simulink model "sg_lens_correct"  (Simulink 8.2)
settings: Solver=VariableStepDiscrete  StartTime=0.0  StopTime=3*Npxl  RelTol=1e-3
values from neighbouring files (symbols this model uses):
  ImgStrmIn = ImgDist'    [tb_lens_correct.m]
  ImgX = SizeI(2)    [tb_lens_correct.m]
  ImgY = SizeI(1)    [tb_lens_correct.m]
  IPM = 0    [tb_lens_correct.m]
  K = 0.00004    (= 4e-05)    [tb_lens_correct.m]
  Npxl = ImgY * ImgX    [tb_lens_correct.m]
  Radius_ROM = Radius'    [tb_lens_correct.m]
  Xcent = (ImgX-1)/2    [tb_lens_correct.m]
  Ycent = (ImgY-1)/2    [tb_lens_correct.m]
libraries: xbsIndex_r4 x87, dspsrcs4 x3
settings Model: Creator=sps  LastModifiedBy=tawassne
settings OptimizationCC: InitFltsAndDblsToZero=on
settings DebuggingCC: SaveWithParameterizedLinksMsg=none  SignalResolutionControl=TryResolveAllWithWarning  SolverPrmCheckMsg=none  MultiTaskDSMMsg=warning  MultiTaskCondExecSysMsg=none
settings RTWCC: IncludeERTFirstTime=on
settings GRTTargetCC: TargetFcnLib=ansi_tfl_tmw.mat

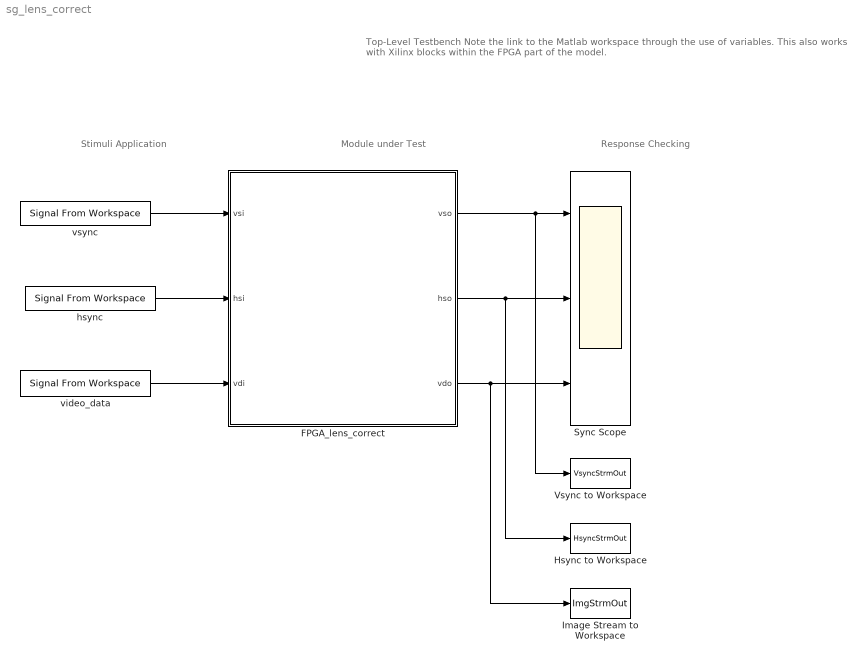
== system sg_lens_correct ==
  note: Top-Level Testbench
      | Note the link to the Matlab workspace through the use of variables.
      | This also works with Xilinx blocks within the FPGA part of the model.
  note: Stimuli Application
  note: Response Checking
  note: Module under Test
  FPGA_lens_correct : Subsystem
  Hsync to Workspace : ToWorkspace  VariableName=HsyncStrmOut  SampleTime=-1
      settings: MaxDataPoints=2*Npxl
  Image Stream to Workspace : ToWorkspace  VariableName=ImgStrmOut  SampleTime=-1
      settings: MaxDataPoints=2*Npxl
  Sync Scope : Scope  NumInputPorts=3
      settings: YMin=-5~-5~-5  YMax=5~5~5
  Vsync to Workspace : ToWorkspace  VariableName=VsyncStrmOut  SampleTime=-1
      settings: MaxDataPoints=2*Npxl
  hsync : dspsrcs4/Signal From Workspace  X=[ zeros(1,ImgX-1) 1 ]  Ts=1  nsamps=1  OutputAfterFinalValue=Cyclic repetition  ignoreOrWarnInputAndFrameLengths=off
  video_data : dspsrcs4/Signal From Workspace  X=[ ImgStrmIn(:) ]  Ts=1  nsamps=1  OutputAfterFinalValue=Cyclic repetition  ignoreOrWarnInputAndFrameLengths=off
  vsync : dspsrcs4/Signal From Workspace  X=[ zeros(1,Npxl-1) 1 ]  Ts=1  nsamps=1  OutputAfterFinalValue=Cyclic repetition  ignoreOrWarnInputAndFrameLengths=off
  wires:
  vsync/1 -> FPGA_lens_correct/1(vsi)
  hsync/1 -> FPGA_lens_correct/2(hsi)
  video_data/1 -> FPGA_lens_correct/3(vdi)
  FPGA_lens_correct/1(vso) -> Sync Scope/1, Vsync to Workspace/1
  FPGA_lens_correct/2(hso) -> Sync Scope/2, Hsync to Workspace/1
  FPGA_lens_correct/3(vdo) -> Sync Scope/3, Image Stream to Workspace/1

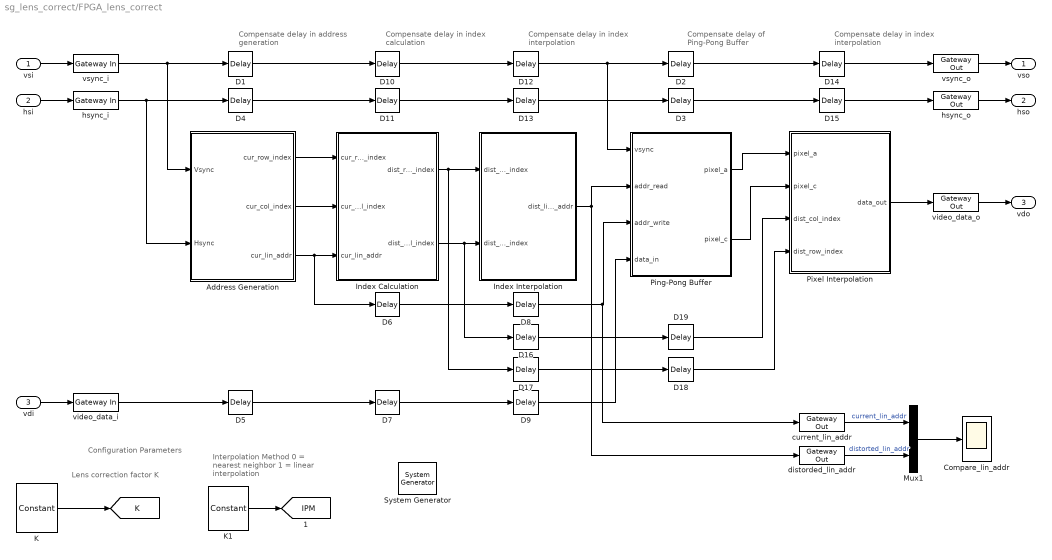
== system sg_lens_correct/FPGA_lens_correct ==
  note: Compensate delay
      | of Ping-Pong Buffer
  note: Compensate delay
      | in index calculation
  note: Compensate delay
      | in index interpolation
  note: Compensate delay
      | in address generation
  note: Configuration Parameters
  note: Lens correction factor K
  note: Interpolation Method
      | 0 = nearest neighbor
      | 1 = linear interpolation
  note: Compensate delay
      | in index interpolation
  vsi : Inport
  hsi : Inport  Port=2
  vdi : Inport  Port=3
  " System Generator" : xbsIndex_r4/ System Generator  Tag=genX  xilinxfamily=spartan6  part=xc6slx150t  speed=-3  package=fgg676  synthesis_tool=XST  clock_wrapper=Clock Enables  directory=./sg_gamma_s6  proj_type=Project Navigator  Synth_file=XST Defaults  Impl_file=ISE Defaults  testbench=off  simulink_period=1  sysclk_period=10  dcm_input_clock_period=10  incr_netlist=off  trim_vbits=Everywhere in SubSystem  dbl_ovrd=According to Block Masks  core_generation=According to Block Masks  run_coregen=off  deprecated_control=off  eval_field=0  block_type=sysgen
      settings: block_version=11.4
  Address Generation : Subsystem
  Compare_lin_addr : Scope
      settings: ShowLegends=on  SaveName=ScopeData3
  D1 : xbsIndex_r4/Delay  rst=off  infoeditControl=Selection of Reset will increase slice count due to use of real FFs and instead of SRLs  en=off  latency=LT_AdrGen  dbl_ovrd=off  reg_retiming=off  block_type=delay
  D{6..7,10..11} (4 alike) : xbsIndex_r4/Delay  rst=off  infoeditControl=Selection of Reset will increase slice count due to use of real FFs and instead of SRLs  en=off  latency=LT_IdxCalc  dbl_ovrd=off  reg_retiming=off  block_type=delay
  D{8..9,12..13,16..17} (6 alike) : xbsIndex_r4/Delay  rst=off  infoeditControl=Selection of Reset will increase slice count due to use of real FFs and instead of SRLs  en=off  latency=LT_IdxInpol  dbl_ovrd=off  reg_retiming=off  block_type=delay
  D14 : xbsIndex_r4/Delay  rst=off  infoeditControl=Selection of Reset will increase slice count due to use of real FFs and instead of SRLs  en=off  latency=LT_PxlInpol  dbl_ovrd=off  reg_retiming=off  block_type=delay
  D15 : xbsIndex_r4/Delay  rst=off  infoeditControl=Selection of Reset will increase slice count due to use of real FFs and instead of SRLs  en=off  latency=LT_PxlInpol  dbl_ovrd=off  reg_retiming=off  block_type=delay
  D{2..3,18..19} (4 alike) : xbsIndex_r4/Delay  rst=off  infoeditControl=Selection of Reset will increase slice count due to use of real FFs and instead of SRLs  en=off  latency=LT_PingPong  dbl_ovrd=off  reg_retiming=off  block_type=delay
  D4 : xbsIndex_r4/Delay  rst=off  infoeditControl=Selection of Reset will increase slice count due to use of real FFs and instead of SRLs  en=off  latency=LT_AdrGen  dbl_ovrd=off  reg_retiming=off  block_type=delay
  D5 : xbsIndex_r4/Delay  rst=off  infoeditControl=Selection of Reset will increase slice count due to use of real FFs and instead of SRLs  en=off  latency=LT_AdrGen  dbl_ovrd=off  reg_retiming=off  block_type=delay
  Index Calculation : Subsystem
  Index Interpolation : Subsystem
  K : xbsIndex_r4/Constant  const=K  gui_display_data_type=Fixed-point  arith_type=Unsigned  n_bits=32  bin_pt=31  preci_type=Single  exp_width=8  frac_width=24  explicit_period=off  period=1  equ=P=C  opselect=C  inp2=PCIN>>17  opr=+  inp1=P  carry=CIN  dbl_ovrd=off  block_type=constant
  K1 : xbsIndex_r4/Constant  const=IPM  gui_display_data_type=Boolean  arith_type=Boolean  n_bits=16  bin_pt=15  preci_type=Single  exp_width=8  frac_width=24  explicit_period=off  period=1  equ=P=C  opselect=C  inp2=PCIN>>17  opr=+  inp1=P  carry=CIN  dbl_ovrd=off  block_type=constant
  Mux1 : Mux  Inputs=2
  Ping-Pong Buffer : Subsystem
  Pixel Interpolation : Subsystem
  current_lin_addr : xbsIndex_r4/Gateway Out  hdl_port=off  timing_constraint=None  locs_specified=off  LOCs={}  block_type=gatewayout
      settings: infoedit="Gateway out block.  Converts Xilinx fixed point or floating-point type inputs into ouputs of type Simulink integer, double, or fixed point.<br><br>Hardware notes:  In hardware these blocks become top level output ports or are discarded, depending on how they are configured."  xl_area=[0, 0, 0, 0, 0, 0, 0]  block_version=VER_STRING_GOES_HERE
  distorded_lin_addr : xbsIndex_r4/Gateway Out  hdl_port=off  timing_constraint=None  locs_specified=off  LOCs={}  block_type=gatewayout
      settings: infoedit="Gateway out block.  Converts Xilinx fixed point or floating-point type inputs into ouputs of type Simulink integer, double, or fixed point.<br><br>Hardware notes:  In hardware these blocks become top level output ports or are discarded, depending on how they are configured."  xl_area=[0, 0, 0, 0, 0, 0, 0]  block_version=VER_STRING_GOES_HERE
  hsync_i : xbsIndex_r4/Gateway In  gui_display_data_type=Fixed-point  arith_type=Boolean  n_bits=1  bin_pt=0  preci_type=Single  exp_width=8  frac_width=24  quantization="Round  (unbiased: +/- Inf)"  overflow=Saturate  period=1  dbl_ovrd=off  timing_constraint=None  locs_specified=off  LOCs={}  hdl_port=on  block_type=gatewayin
      settings: infoedit="Gateway in block.  Converts inputs of type Simulink integer, double and fixed point to  Xilinx fixed point type.<br><br>Hardware notes:  In hardware these blocks become top level input ports."  xl_area=[0, 0, 0, 0, 0, 0, 0]  block_version=VER_STRING_GOES_HERE
  hsync_o : xbsIndex_r4/Gateway Out  hdl_port=on  timing_constraint=None  locs_specified=off  LOCs={}  block_type=gatewayout
      settings: infoedit="Gateway out block.  Converts Xilinx fixed point inputs into ouputs of type Simulink integer, double, or fixed point.<P><P>Hardware notes:  In hardware these blocks become top level output ports or are discarded, depending on how they are configured."  xl_area=[0, 0, 0, 0, 0, 0, 0]  block_version=VER_STRING_GOES_HERE
  video_data_i : xbsIndex_r4/Gateway In  gui_display_data_type=Fixed-point  arith_type=Unsigned  n_bits=8  bin_pt=0  preci_type=Single  exp_width=8  frac_width=24  quantization="Round  (unbiased: +/- Inf)"  overflow=Saturate  period=1  dbl_ovrd=off  timing_constraint=None  locs_specified=off  LOCs={}  hdl_port=on  block_type=gatewayin
      settings: infoedit="Gateway in block.  Converts inputs of type Simulink integer, double and fixed point to  Xilinx fixed point type.<br><br>Hardware notes:  In hardware these blocks become top level input ports."  xl_area=[0, 0, 0, 0, 0, 0, 0]  block_version=VER_STRING_GOES_HERE
  video_data_o : xbsIndex_r4/Gateway Out  hdl_port=on  timing_constraint=None  locs_specified=off  LOCs={}  block_type=gatewayout
      settings: infoedit="Gateway out block.  Converts Xilinx fixed point inputs into ouputs of type Simulink integer, double, or fixed point.<P><P>Hardware notes:  In hardware these blocks become top level output ports or are discarded, depending on how they are configured."  xl_area=[0, 0, 0, 0, 0, 0, 0]  block_version=VER_STRING_GOES_HERE
  vsync_i : xbsIndex_r4/Gateway In  gui_display_data_type=Fixed-point  arith_type=Boolean  n_bits=1  bin_pt=0  preci_type=Single  exp_width=8  frac_width=24  quantization="Round  (unbiased: +/- Inf)"  overflow=Saturate  period=1  dbl_ovrd=off  timing_constraint=None  locs_specified=off  LOCs={}  hdl_port=on  block_type=gatewayin
      settings: infoedit="Gateway in block.  Converts inputs of type Simulink integer, double and fixed point to  Xilinx fixed point type.<br><br>Hardware notes:  In hardware these blocks become top level input ports."  xl_area=[0, 0, 0, 0, 0, 0, 0]  block_version=VER_STRING_GOES_HERE
  vsync_o : xbsIndex_r4/Gateway Out  hdl_port=on  timing_constraint=None  locs_specified=off  LOCs={}  block_type=gatewayout
      settings: infoedit="Gateway out block.  Converts Xilinx fixed point inputs into ouputs of type Simulink integer, double, or fixed point.<P><P>Hardware notes:  In hardware these blocks become top level output ports or are discarded, depending on how they are configured."  xl_area=[0, 0, 0, 0, 0, 0, 0]  block_version=VER_STRING_GOES_HERE
  vso : Outport
  hso : Outport  Port=2
  vdo : Outport  Port=3
  tag scope: IPM=global, K=global
  wires:
  vdi/1 -> video_data_i/1
  video_data_o/1 -> vdo/1
  vsi/1 -> vsync_i/1
  hsi/1 -> hsync_i/1
  vsync_o/1 -> vso/1
  hsync_o/1 -> hso/1
  vsync_i/1 -> Address Generation/1(Vsync), D1/1
  hsync_i/1 -> Address Generation/2(Hsync), D4/1
  Address Generation/3(cur_lin_addr) -> Index Calculation/3(cur_lin_addr), D6/1
  D2/1 -> D14/1
  D3/1 -> D15/1
  video_data_i/1 -> D5/1
  Address Generation/1(cur_row_index) -> Index Calculation/1(cur_row_index)
  Address Generation/2(cur_col_index) -> Index Calculation/2(cur_col_index)
  Index Interpolation/1(dist_lin_addr) -> Ping-Pong Buffer/2(addr_read), distorded_lin_addr/1
  Index Calculation/1(dist_row_index) -> Index Interpolation/1(dist_row_index), D17/1
  Index Calculation/2(dist_col_index) -> Index Interpolation/2(dist_col_index), D16/1
  current_lin_addr/1 -> Mux1/1  "current_lin_addr"
  distorded_lin_addr/1 -> Mux1/2  "distorted_lin_addr"
  Mux1/1 -> Compare_lin_addr/1
  D1/1 -> D10/1
  D4/1 -> D11/1
  D5/1 -> D7/1
  D7/1 -> D9/1
  D6/1 -> D8/1
  D10/1 -> D12/1
  D11/1 -> D13/1
  D12/1 -> D2/1, Ping-Pong Buffer/1(vsync)
  D13/1 -> D3/1
  D8/1 -> current_lin_addr/1, Ping-Pong Buffer/3(addr_write)
  D9/1 -> Ping-Pong Buffer/4(data_in)
  K/1 -> [K]
  K1/1 -> [IPM]
  D14/1 -> vsync_o/1
  D15/1 -> hsync_o/1
  D16/1 -> D19/1
  D17/1 -> D18/1
  Pixel Interpolation/1(data_out) -> video_data_o/1
  D19/1 -> Pixel Interpolation/3(dist_col_index)
  D18/1 -> Pixel Interpolation/4(dist_row_index)
  Ping-Pong Buffer/1(pixel_a) -> Pixel Interpolation/1(pixel_a)
  Ping-Pong Buffer/2(pixel_c) -> Pixel Interpolation/2(pixel_c)

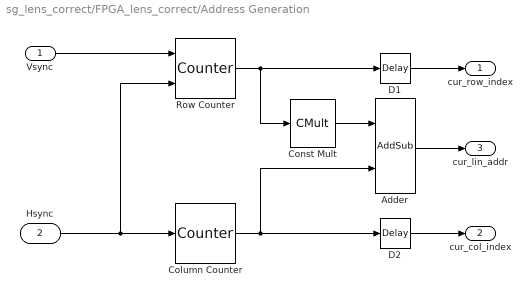
== system sg_lens_correct/FPGA_lens_correct/Address Generation ==
  Vsync : Inport
  Hsync : Inport  Port=2
  Adder : xbsIndex_r4/AddSub  mode=Addition  use_carryin=off  use_carryout=off  en=off  latency=1  precision=User Defined  arith_type=Unsigned  n_bits=ceil(log2(Npxl))  bin_pt=0  quantization=Truncate  overflow=Wrap  dbl_ovrd=off  use_behavioral_HDL=off  hw_selection=Fabric  pipelined=off  block_type=addsub
  Column Counter : xbsIndex_r4/Counter  cnt_type=Count Limited  cnt_to=ImgX-1  operation=Up  start_count=0  cnt_by_val=1  arith_type=Unsigned  n_bits=ceil(log2(ImgX))  bin_pt=0  load_pin=off  rst=on  en=off  explicit_period=on  period=1  dbl_ovrd=off  use_behavioral_HDL=off  implementation=Fabric  block_type=counter
  Const Mult : xbsIndex_r4/CMult  const=ImgX  gui_display_data_type=Fixed-point  const_n_bits=ceil(log2(ImgX+1))  const_bin_pt=0  float_type=Single  exp_bits=8  fraction_bits=24  en=off  latency=0  precision=Full  arith_type=Unsigned  n_bits=16  bin_pt=0  quantization=Truncate  overflow=Wrap  dbl_ovrd=off  use_behavioral_HDL=off  mem_type=Distributed RAM  pipeline=off  block_type=cmult
  D1 : xbsIndex_r4/Delay  rst=off  infoeditControl=Selection of Reset will increase slice count due to use of real FFs and instead of SRLs  en=off  latency=1  dbl_ovrd=off  reg_retiming=off  block_type=delay
  D2 : xbsIndex_r4/Delay  rst=off  infoeditControl=Selection of Reset will increase slice count due to use of real FFs and instead of SRLs  en=off  latency=1  dbl_ovrd=off  reg_retiming=off  block_type=delay
  Row Counter : xbsIndex_r4/Counter  cnt_type=Count Limited  cnt_to=ImgY-1  operation=Up  start_count=0  cnt_by_val=1  arith_type=Unsigned  n_bits=ceil(log2(ImgY))  bin_pt=0  load_pin=off  rst=on  en=on  explicit_period=on  period=1  dbl_ovrd=off  use_behavioral_HDL=off  implementation=Fabric  block_type=counter
  cur_row_index : Outport
  cur_col_index : Outport  Port=2
  cur_lin_addr : Outport  Port=3
  wires:
  Column Counter/1 -> Adder/2, D2/1
  Row Counter/1 -> Const Mult/1, D1/1
  Const Mult/1 -> Adder/1
  Vsync/1 -> Row Counter/1
  Adder/1 -> cur_lin_addr/1
  Hsync/1 -> Column Counter/1, Row Counter/2
  D1/1 -> cur_row_index/1
  D2/1 -> cur_col_index/1

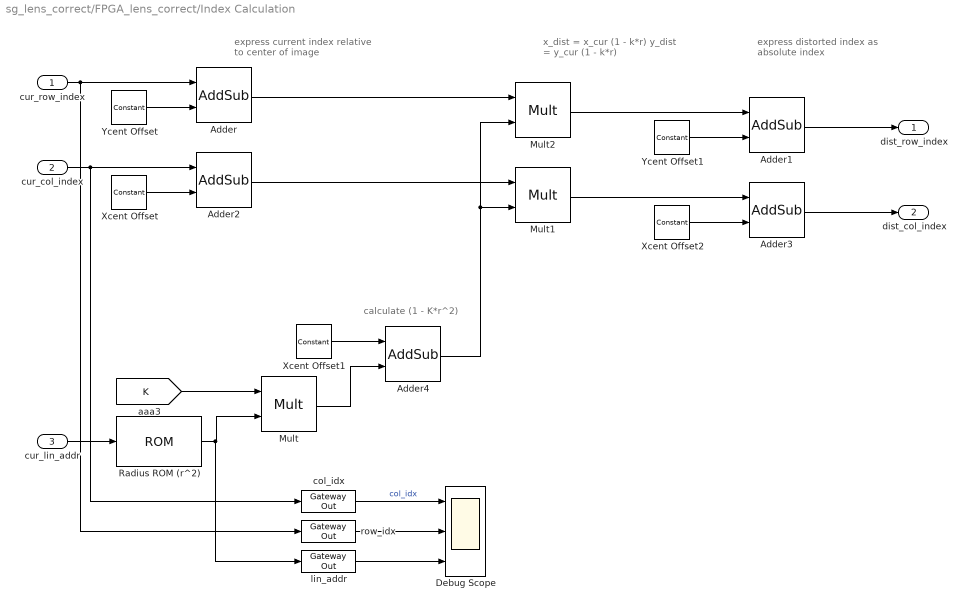
== system sg_lens_correct/FPGA_lens_correct/Index Calculation ==
  note: express current index
      | relative to center of image
  note: calculate (1 - K*r^2)
  note: x_dist = x_cur (1 - k*r)
      | y_dist = y_cur (1 - k*r)
  note: express distorted index
      | as absolute index
  cur_row_index : Inport
  cur_col_index : Inport  Port=2
  cur_lin_addr : Inport  Port=3
  Adder : xbsIndex_r4/AddSub  mode=Subtraction  use_carryin=off  use_carryout=off  en=off  latency=5  precision=User Defined  arith_type="Signed  (2's comp)"  n_bits=ceil(log2(ImgY))+1  bin_pt=1  quantization=Truncate  overflow=Wrap  dbl_ovrd=off  use_behavioral_HDL=off  hw_selection=Fabric  pipelined=off  block_type=addsub
  Adder1 : xbsIndex_r4/AddSub  mode=Addition  use_carryin=off  use_carryout=off  en=off  latency=1  precision=User Defined  arith_type=Unsigned  n_bits=ceil(log2(ImgY))+15  bin_pt=15  quantization="Round  (unbiased: +/- Inf)"  overflow=Wrap  dbl_ovrd=off  use_behavioral_HDL=off  hw_selection=Fabric  pipelined=off  block_type=addsub
  Adder2 : xbsIndex_r4/AddSub  mode=Subtraction  use_carryin=off  use_carryout=off  en=off  latency=5  precision=User Defined  arith_type="Signed  (2's comp)"  n_bits=ceil(log2(ImgX))+1  bin_pt=1  quantization=Truncate  overflow=Wrap  dbl_ovrd=off  use_behavioral_HDL=off  hw_selection=Fabric  pipelined=off  block_type=addsub
  Adder3 : xbsIndex_r4/AddSub  mode=Addition  use_carryin=off  use_carryout=off  en=off  latency=1  precision=User Defined  arith_type=Unsigned  n_bits=ceil(log2(ImgX))+15  bin_pt=15  quantization="Round  (unbiased: +/- Inf)"  overflow=Wrap  dbl_ovrd=off  use_behavioral_HDL=off  hw_selection=Fabric  pipelined=off  block_type=addsub
  Adder4 : xbsIndex_r4/AddSub  mode=Subtraction  use_carryin=off  use_carryout=off  en=off  latency=1  precision=Full  arith_type="Signed  (2's comp)"  n_bits=ceil(log2(ImgX))+1  bin_pt=1  quantization=Truncate  overflow=Wrap  dbl_ovrd=off  use_behavioral_HDL=off  hw_selection=Fabric  pipelined=off  block_type=addsub
  Debug Scope : Scope  NumInputPorts=3
      settings: ShowLegends=on  YMin=0~0~0  YMax=100~100~5000
  Mult : xbsIndex_r4/Mult  precision=Full  arith_type="Signed  (2's comp)"  n_bits=16  bin_pt=14  quantization=Truncate  overflow=Wrap  en=off  latency=3  dbl_ovrd=off  use_behavioral_HDL=off  opt=Speed  use_embedded=on  optimum_pipeline=off  pipeline=on  use_rpm=on  placement_style=Triangular  block_type=mult
  Mult1 : xbsIndex_r4/Mult  precision=Full  arith_type="Signed  (2's comp)"  n_bits=16  bin_pt=14  quantization=Truncate  overflow=Wrap  en=off  latency=3  dbl_ovrd=off  use_behavioral_HDL=off  opt=Speed  use_embedded=on  optimum_pipeline=off  pipeline=on  use_rpm=on  placement_style=Triangular  block_type=mult
  Mult2 : xbsIndex_r4/Mult  precision=Full  arith_type="Signed  (2's comp)"  n_bits=16  bin_pt=14  quantization=Truncate  overflow=Wrap  en=off  latency=3  dbl_ovrd=off  use_behavioral_HDL=off  opt=Speed  use_embedded=on  optimum_pipeline=off  pipeline=on  use_rpm=on  placement_style=Triangular  block_type=mult
  Radius ROM (r^2) : xbsIndex_r4/ROM  depth=Npxl  initVector=Radius_ROM  distributed_mem=Block RAM  rst=off  init_reg=0  en=off  latency=1  gui_display_data_type=Fixed-point  arith_type=Unsigned  n_bits=ceil(log2(max(max(Radius_ROM))+1)) + 1  bin_pt=1  preci_type=Single  exp_width=8  frac_width=24  dbl_ovrd=off  optimize=Area  use_rpm=on  block_type=sprom
  Xcent Offset : xbsIndex_r4/Constant  const=Xcent  gui_display_data_type=Fixed-point  arith_type=Unsigned  n_bits=ceil(log2(ImgX))  bin_pt=1  preci_type=Single  exp_width=8  frac_width=24  explicit_period=off  period=1  equ=P=C  opselect=C  inp2=PCIN>>17  opr=+  inp1=P  carry=CIN  dbl_ovrd=off  block_type=constant
  Xcent Offset1 : xbsIndex_r4/Constant  const=1  gui_display_data_type=Fixed-point  arith_type=Unsigned  n_bits=1  bin_pt=0  preci_type=Single  exp_width=8  frac_width=24  explicit_period=off  period=1  equ=P=C  opselect=C  inp2=PCIN>>17  opr=+  inp1=P  carry=CIN  dbl_ovrd=off  block_type=constant
  Xcent Offset2 : xbsIndex_r4/Constant  const=Xcent  gui_display_data_type=Fixed-point  arith_type=Unsigned  n_bits=ceil(log2(ImgX))  bin_pt=1  preci_type=Single  exp_width=8  frac_width=24  explicit_period=off  period=1  equ=P=C  opselect=C  inp2=PCIN>>17  opr=+  inp1=P  carry=CIN  dbl_ovrd=off  block_type=constant
  Ycent Offset : xbsIndex_r4/Constant  const=Ycent  gui_display_data_type=Fixed-point  arith_type=Unsigned  n_bits=ceil(log2(ImgY))  bin_pt=1  preci_type=Single  exp_width=8  frac_width=24  explicit_period=off  period=1  equ=P=C  opselect=C  inp2=PCIN>>17  opr=+  inp1=P  carry=CIN  dbl_ovrd=off  block_type=constant
  Ycent Offset1 : xbsIndex_r4/Constant  const=Ycent  gui_display_data_type=Fixed-point  arith_type=Unsigned  n_bits=ceil(log2(ImgY))  bin_pt=1  preci_type=Single  exp_width=8  frac_width=24  explicit_period=off  period=1  equ=P=C  opselect=C  inp2=PCIN>>17  opr=+  inp1=P  carry=CIN  dbl_ovrd=off  block_type=constant
  col_idx : xbsIndex_r4/Gateway Out  hdl_port=off  timing_constraint=None  locs_specified=off  LOCs={}  block_type=gatewayout
      settings: infoedit="Gateway out block.  Converts Xilinx fixed point or floating-point type inputs into ouputs of type Simulink integer, double, or fixed point.<br><br>Hardware notes:  In hardware these blocks become top level output ports or are discarded, depending on how they are configured."  xl_area=[0, 0, 0, 0, 0, 0, 0]  block_version=VER_STRING_GOES_HERE
  lin_addr : xbsIndex_r4/Gateway Out  hdl_port=off  timing_constraint=None  locs_specified=off  LOCs={}  block_type=gatewayout
      settings: infoedit="Gateway out block.  Converts Xilinx fixed point or floating-point type inputs into ouputs of type Simulink integer, double, or fixed point.<br><br>Hardware notes:  In hardware these blocks become top level output ports or are discarded, depending on how they are configured."  xl_area=[0, 0, 0, 0, 0, 0, 0]  block_version=VER_STRING_GOES_HERE
  row_idx : xbsIndex_r4/Gateway Out  hdl_port=off  timing_constraint=None  locs_specified=off  LOCs={}  block_type=gatewayout
      settings: infoedit="Gateway out block.  Converts Xilinx fixed point or floating-point type inputs into ouputs of type Simulink integer, double, or fixed point.<br><br>Hardware notes:  In hardware these blocks become top level output ports or are discarded, depending on how they are configured."  xl_area=[0, 0, 0, 0, 0, 0, 0]  block_version=VER_STRING_GOES_HERE
  dist_row_index : Outport
  dist_col_index : Outport  Port=2
  wires:
  cur_lin_addr/1 -> Radius ROM (r^2)/1
  Radius ROM (r^2)/1 -> lin_addr/1, Mult/2
  cur_row_index/1 -> row_idx/1, Adder/1
  Ycent Offset/1 -> Adder/2
  Xcent Offset/1 -> Adder2/2
  cur_col_index/1 -> col_idx/1, Adder2/1
  Mult/1 -> Adder4/2
  Xcent Offset1/1 -> Adder4/1
  Adder2/1 -> Mult1/1
  Adder4/1 -> Mult2/2, Mult1/2
  Adder/1 -> Mult2/1
  Ycent Offset1/1 -> Adder1/2
  Xcent Offset2/1 -> Adder3/2
  Mult2/1 -> Adder1/1
  Adder1/1 -> dist_row_index/1
  Mult1/1 -> Adder3/1
  Adder3/1 -> dist_col_index/1
  [K] -> Mult/1
  col_idx/1 -> Debug Scope/1  "col_idx"
  row_idx/1 -> Debug Scope/2
  lin_addr/1 -> Debug Scope/3

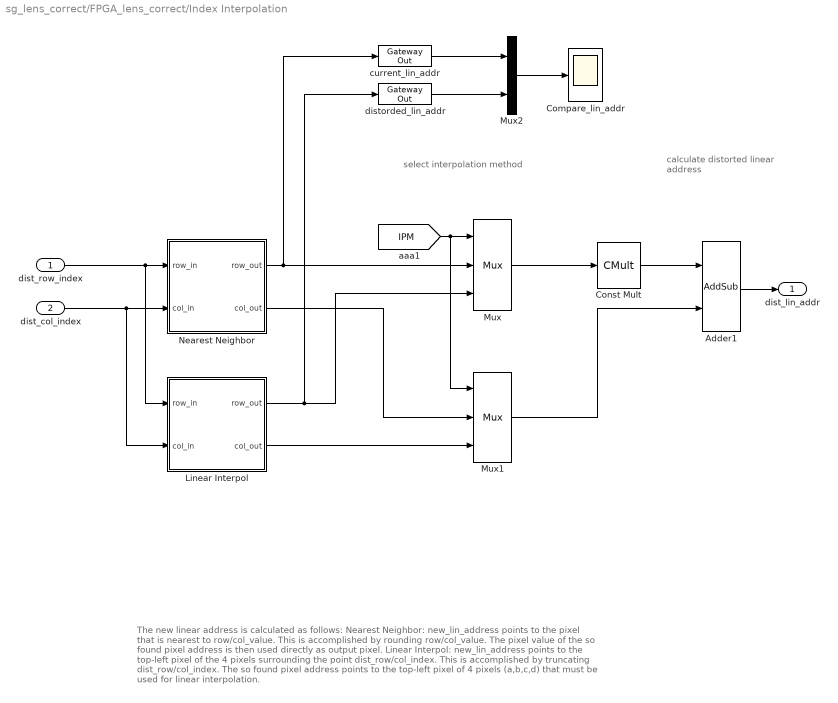
== system sg_lens_correct/FPGA_lens_correct/Index Interpolation ==
  note: calculate distorted
      | linear address
  note: select interpolation method
  note: The new linear address is calculated as follows:
      |
      | Nearest Neighbor:
      |   new_lin_address points to the pixel that is nearest to row/col_value. This is accomplished
      |   by rounding row/col_value. The pixel value of the so found pixel address is then used directly
      |   as output pixel.
      |
      | Linear Interpol:
      |   new_lin_address points to the top-left pixel of the 4 pixels surrounding the point dist_row/col_index.
      |   This is accomplished by truncating dist_row/col_index. The so found pixel address points to the
      |   top-left pixel of 4 pixels (a,b,c,d) that must be used for linear interpolation.
  dist_row_index : Inport
  dist_col_index : Inport  Port=2
  Adder1 : xbsIndex_r4/AddSub  mode=Addition  use_carryin=off  use_carryout=off  en=off  latency=1  precision=User Defined  arith_type=Unsigned  n_bits=ceil(log2(Npxl))  bin_pt=0  quantization="Round  (unbiased: +/- Inf)"  overflow=Saturate  dbl_ovrd=off  use_behavioral_HDL=off  hw_selection=Fabric  pipelined=off  block_type=addsub
  Compare_lin_addr : Scope
      settings: ShowLegends=on  SaveName=ScopeData2
  Const Mult : xbsIndex_r4/CMult  const=ImgX  gui_display_data_type=Fixed-point  const_n_bits=ceil(log2(ImgX+1))  const_bin_pt=0  float_type=Single  exp_bits=8  fraction_bits=24  en=off  latency=0  precision=Full  arith_type="Signed  (2's comp)"  n_bits=16  bin_pt=14  quantization=Truncate  overflow=Wrap  dbl_ovrd=off  use_behavioral_HDL=off  mem_type=Distributed RAM  pipeline=off  block_type=cmult
  Linear Interpol : Subsystem
  Mux : xbsIndex_r4/Mux  inputs=2  en=off  latency=1  precision=Full  arith_type=Unsigned  n_bits=16  bin_pt=14  quantization=Truncate  overflow=Wrap  dbl_ovrd=off  block_type=mux
  Mux1 : xbsIndex_r4/Mux  inputs=2  en=off  latency=1  precision=Full  arith_type=Unsigned  n_bits=16  bin_pt=14  quantization=Truncate  overflow=Wrap  dbl_ovrd=off  block_type=mux
  Mux2 : Mux  Inputs=2
  Nearest Neighbor : Subsystem
  current_lin_addr : xbsIndex_r4/Gateway Out  hdl_port=off  timing_constraint=None  locs_specified=off  LOCs={}  block_type=gatewayout
      settings: infoedit="Gateway out block.  Converts Xilinx fixed point or floating-point type inputs into ouputs of type Simulink integer, double, or fixed point.<br><br>Hardware notes:  In hardware these blocks become top level output ports or are discarded, depending on how they are configured."  xl_area=[0, 0, 0, 0, 0, 0, 0]  block_version=VER_STRING_GOES_HERE
  distorded_lin_addr : xbsIndex_r4/Gateway Out  hdl_port=off  timing_constraint=None  locs_specified=off  LOCs={}  block_type=gatewayout
      settings: infoedit="Gateway out block.  Converts Xilinx fixed point or floating-point type inputs into ouputs of type Simulink integer, double, or fixed point.<br><br>Hardware notes:  In hardware these blocks become top level output ports or are discarded, depending on how they are configured."  xl_area=[0, 0, 0, 0, 0, 0, 0]  block_version=VER_STRING_GOES_HERE
  dist_lin_addr : Outport
  wires:
  Const Mult/1 -> Adder1/1
  dist_row_index/1 -> Nearest Neighbor/1(row_in), Linear Interpol/1(row_in)
  dist_col_index/1 -> Nearest Neighbor/2(col_in), Linear Interpol/2(col_in)
  Nearest Neighbor/1(row_out) -> current_lin_addr/1, Mux/2
  Linear Interpol/1(row_out) -> distorded_lin_addr/1, Mux/3
  Linear Interpol/2(col_out) -> Mux1/3
  Nearest Neighbor/2(col_out) -> Mux1/2
  Mux/1 -> Const Mult/1
  Mux1/1 -> Adder1/2
  [IPM] -> Mux/1, Mux1/1
  Adder1/1 -> dist_lin_addr/1
  current_lin_addr/1 -> Mux2/1
  distorded_lin_addr/1 -> Mux2/2
  Mux2/1 -> Compare_lin_addr/1

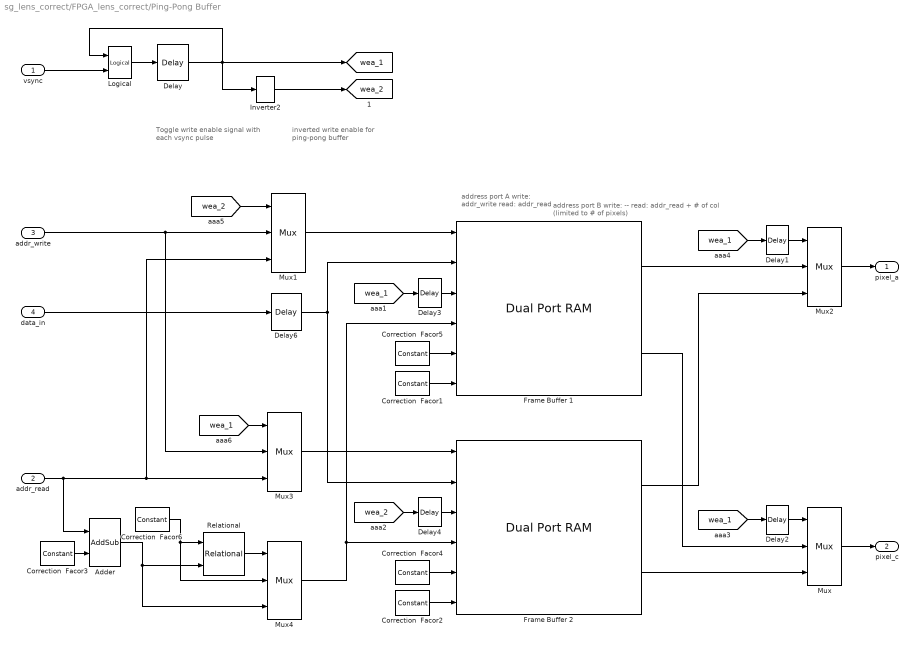
== system sg_lens_correct/FPGA_lens_correct/Ping-Pong Buffer ==
  note: Toggle write enable signal
      | with each vsync pulse
  note: inverted write enable
      | for ping-pong buffer
  note: address port B
      | write: --
      | read: addr_read + # of col (limited to # of pixels)
  note: address port A
      | write: addr_write
      | read: addr_read
  vsync : Inport
  addr_read : Inport  Port=2
  addr_write : Inport  Port=3
  data_in : Inport  Port=4
  Adder : xbsIndex_r4/AddSub  mode=Addition  use_carryin=off  use_carryout=off  en=off  latency=0  precision=User Defined  arith_type=Unsigned  n_bits=ceil(log2(Npxl))  bin_pt=0  quantization=Truncate  overflow=Saturate  dbl_ovrd=off  use_behavioral_HDL=off  hw_selection=Fabric  pipelined=off  block_type=addsub
  Correction  Facor1 : xbsIndex_r4/Constant  const=0  gui_display_data_type=Fixed-point  arith_type=Boolean  n_bits=16  bin_pt=15  preci_type=Single  exp_width=8  frac_width=24  explicit_period=off  period=1  equ=P=C  opselect=C  inp2=PCIN>>17  opr=+  inp1=P  carry=CIN  dbl_ovrd=off  block_type=constant
  Correction  Facor2 : xbsIndex_r4/Constant  const=0  gui_display_data_type=Fixed-point  arith_type=Boolean  n_bits=16  bin_pt=15  preci_type=Single  exp_width=8  frac_width=24  explicit_period=off  period=1  equ=P=C  opselect=C  inp2=PCIN>>17  opr=+  inp1=P  carry=CIN  dbl_ovrd=off  block_type=constant
  Correction  Facor3 : xbsIndex_r4/Constant  const=ImgX  gui_display_data_type=Fixed-point  arith_type=Unsigned  n_bits=ceil(log2(ImgX))+1  bin_pt=0  preci_type=Single  exp_width=8  frac_width=24  explicit_period=off  period=1  equ=P=C  opselect=C  inp2=PCIN>>17  opr=+  inp1=P  carry=CIN  dbl_ovrd=off  block_type=constant
  Correction  Facor4 : xbsIndex_r4/Constant  const=0  gui_display_data_type=Fixed-point  arith_type=Unsigned  n_bits=8  bin_pt=0  preci_type=Single  exp_width=8  frac_width=24  explicit_period=off  period=1  equ=P=C  opselect=C  inp2=PCIN>>17  opr=+  inp1=P  carry=CIN  dbl_ovrd=off  block_type=constant
  Correction  Facor5 : xbsIndex_r4/Constant  const=0  gui_display_data_type=Fixed-point  arith_type=Unsigned  n_bits=8  bin_pt=0  preci_type=Single  exp_width=8  frac_width=24  explicit_period=off  period=1  equ=P=C  opselect=C  inp2=PCIN>>17  opr=+  inp1=P  carry=CIN  dbl_ovrd=off  block_type=constant
  Correction  Facor6 : xbsIndex_r4/Constant  const=Npxl-1  gui_display_data_type=Fixed-point  arith_type=Unsigned  n_bits=ceil(log2(Npxl))  bin_pt=0  preci_type=Single  exp_width=8  frac_width=24  explicit_period=off  period=1  equ=P=C  opselect=C  inp2=PCIN>>17  opr=+  inp1=P  carry=CIN  dbl_ovrd=off  block_type=constant
  Delay{,3..4,6} (4 alike) : xbsIndex_r4/Delay  rst=off  infoeditControl=Selection of Reset will increase slice count due to use of real FFs and instead of SRLs  en=off  latency=1  dbl_ovrd=off  reg_retiming=off  block_type=delay
  Delay1 : xbsIndex_r4/Delay  rst=off  infoeditControl=Selection of Reset will increase slice count due to use of real FFs and instead of SRLs  en=off  latency=2  dbl_ovrd=off  reg_retiming=off  block_type=delay
  Delay2 : xbsIndex_r4/Delay  rst=off  infoeditControl=Selection of Reset will increase slice count due to use of real FFs and instead of SRLs  en=off  latency=2  dbl_ovrd=off  reg_retiming=off  block_type=delay
  Frame Buffer 1 : xbsIndex_r4/Dual Port RAM  depth=2^(ceil(log2(Npxl)))  initVector=1*ones(1,Npxl)  distributed_mem=Block RAM  init_a=0  init_b=0  rst_a=off  rst_b=off  en_a=off  en_b=off  latency=1  write_mode_A=No Read On Write  write_mode_B=No Read On Write  dbl_ovrd=off  optimize=Area  use_rpm=on  block_type=dpram
  Frame Buffer 2 : xbsIndex_r4/Dual Port RAM  depth=2^(ceil(log2(Npxl)))  initVector=1*ones(1,Npxl)  distributed_mem=Block RAM  init_a=0  init_b=0  rst_a=off  rst_b=off  en_a=off  en_b=off  latency=1  write_mode_A=No Read On Write  write_mode_B=No Read On Write  dbl_ovrd=off  optimize=Area  use_rpm=on  block_type=dpram
  Inverter2 : xbsIndex_r4/Inverter  en=off  latency=0  dbl_ovrd=off  block_type=inv
  Logical : xbsIndex_r4/Logical  logical_function=XOR  inputs=2  en=off  latency=0  precision=Full  arith_type=Unsigned  n_bits=16  bin_pt=0  align_bp=on  dbl_ovrd=off  block_type=logical
  Mux : xbsIndex_r4/Mux  inputs=2  en=off  latency=0  precision=Full  arith_type=Unsigned  n_bits=16  bin_pt=14  quantization=Truncate  overflow=Wrap  dbl_ovrd=off  block_type=mux
  Mux1 : xbsIndex_r4/Mux  inputs=2  en=off  latency=1  precision=Full  arith_type=Unsigned  n_bits=16  bin_pt=14  quantization=Truncate  overflow=Wrap  dbl_ovrd=off  block_type=mux
  Mux2 : xbsIndex_r4/Mux  inputs=2  en=off  latency=0  precision=Full  arith_type=Unsigned  n_bits=16  bin_pt=14  quantization=Truncate  overflow=Wrap  dbl_ovrd=off  block_type=mux
  Mux3 : xbsIndex_r4/Mux  inputs=2  en=off  latency=1  precision=Full  arith_type=Unsigned  n_bits=16  bin_pt=14  quantization=Truncate  overflow=Wrap  dbl_ovrd=off  block_type=mux
  Mux4 : xbsIndex_r4/Mux  inputs=2  en=off  latency=1  precision=Full  arith_type=Unsigned  n_bits=16  bin_pt=14  quantization=Truncate  overflow=Wrap  dbl_ovrd=off  block_type=mux
  Relational : xbsIndex_r4/Relational  mode=a>=b  en=off  latency=0  dbl_ovrd=off  block_type=relational
  pixel_a : Outport
  pixel_c : Outport  Port=2
  tag scope: wea_1=global, wea_2=global
  wires:
  [wea_1] -> Delay3/1
  Correction  Facor1/1 -> Frame Buffer 1/6
  Correction  Facor2/1 -> Frame Buffer 2/6
  Correction  Facor4/1 -> Frame Buffer 2/5
  Correction  Facor5/1 -> Frame Buffer 1/5
  Mux/1 -> pixel_c/1
  Frame Buffer 2/2 -> Mux/3
  Frame Buffer 1/2 -> Mux/2
  [wea_1] -> Delay2/1
  Inverter2/1 -> [wea_2]
  [wea_2] -> Delay4/1
  Logical/1 -> Delay/1
  Delay/1 -> Logical/1, Inverter2/1, [wea_1]
  vsync/1 -> Logical/2
  Delay2/1 -> Mux/1
  [wea_1] -> Delay1/1
  Delay1/1 -> Mux2/1
  Frame Buffer 1/1 -> Mux2/2
  Mux2/1 -> pixel_a/1
  Frame Buffer 2/1 -> Mux2/3
  addr_read/1 -> Adder/1, Mux3/3, Mux1/3
  Correction  Facor3/1 -> Adder/2
  addr_write/1 -> Mux3/2, Mux1/2
  Mux1/1 -> Frame Buffer 1/1
  Mux3/1 -> Frame Buffer 2/1
  data_in/1 -> Delay6/1
  Delay6/1 -> Frame Buffer 2/2, Frame Buffer 1/2
  Adder/1 -> Relational/2, Mux4/3
  Correction  Facor6/1 -> Relational/1, Mux4/2
  Relational/1 -> Mux4/1
  Mux4/1 -> Frame Buffer 2/4, Frame Buffer 1/4
  [wea_2] -> Mux1/1
  [wea_1] -> Mux3/1
  Delay3/1 -> Frame Buffer 1/3
  Delay4/1 -> Frame Buffer 2/3

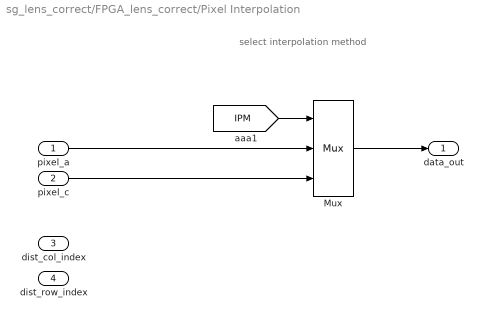
== system sg_lens_correct/FPGA_lens_correct/Pixel Interpolation ==
  note: select interpolation method
  pixel_a : Inport
  pixel_c : Inport  Port=2
  dist_col_index : Inport  Port=3
  dist_row_index : Inport  Port=4
  Mux : xbsIndex_r4/Mux  inputs=2  en=off  latency=1  precision=Full  arith_type=Unsigned  n_bits=16  bin_pt=14  quantization=Truncate  overflow=Wrap  dbl_ovrd=off  block_type=mux
  data_out : Outport
  wires:
  [IPM] -> Mux/1
  Mux/1 -> data_out/1
  pixel_a/1 -> Mux/2
  pixel_c/1 -> Mux/3

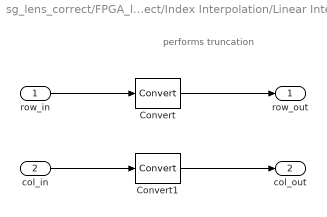
== system sg_lens_correct/FPGA_lens_correct/Index Interpolation/Linear Interpol ==
  note: performs truncation
  row_in : Inport
  col_in : Inport  Port=2
  Convert : xbsIndex_r4/Convert  gui_display_data_type=Fixed-point  arith_type=Unsigned  n_bits=ceil(log2(ImgY))  bin_pt=0  float_type=Single  exp_bits=8  fraction_bits=24  quantization=Truncate  overflow=Saturate  en=off  latency=1  dbl_ovrd=off  pipeline=off  block_type=convert
  Convert1 : xbsIndex_r4/Convert  gui_display_data_type=Fixed-point  arith_type=Unsigned  n_bits=ceil(log2(ImgX))  bin_pt=0  float_type=Single  exp_bits=8  fraction_bits=24  quantization=Truncate  overflow=Saturate  en=off  latency=1  dbl_ovrd=off  pipeline=off  block_type=convert
  row_out : Outport
  col_out : Outport  Port=2
  wires:
  row_in/1 -> Convert/1
  Convert/1 -> row_out/1
  col_in/1 -> Convert1/1
  Convert1/1 -> col_out/1

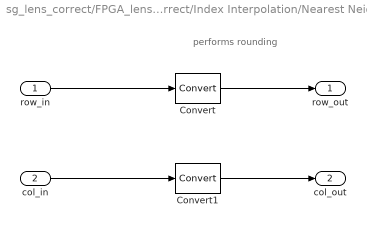
== system sg_lens_correct/FPGA_lens_correct/Index Interpolation/Nearest Neighbor ==
  note: performs rounding
  row_in : Inport
  col_in : Inport  Port=2
  Convert : xbsIndex_r4/Convert  gui_display_data_type=Fixed-point  arith_type=Unsigned  n_bits=ceil(log2(ImgY))  bin_pt=0  float_type=Single  exp_bits=8  fraction_bits=24  quantization="Round  (unbiased: +/- Inf)"  overflow=Saturate  en=off  latency=1  dbl_ovrd=off  pipeline=off  block_type=convert
  Convert1 : xbsIndex_r4/Convert  gui_display_data_type=Fixed-point  arith_type=Unsigned  n_bits=ceil(log2(ImgX))  bin_pt=0  float_type=Single  exp_bits=8  fraction_bits=24  quantization="Round  (unbiased: +/- Inf)"  overflow=Saturate  en=off  latency=1  dbl_ovrd=off  pipeline=off  block_type=convert
  row_out : Outport
  col_out : Outport  Port=2
  wires:
  Convert/1 -> row_out/1
  Convert1/1 -> col_out/1
  row_in/1 -> Convert/1
  col_in/1 -> Convert1/1
